simulink model "fazova_trajektorie"  (R2018a)
settings: Solver=VariableStepAuto  StartTime=0.0  StopTime=20  RelTol=1e-3
values from neighbouring files (symbols this model uses):
  K2 = 0.02    [init.m]
  Kz = 20    [init.m]
  T = 2    [init.m]
  Ul = 10    [init.m]
  Un = 25    [init.m]
  w0 = w(i)    [init.m]
settings Model: Creator=vejvarm  LastModifiedBy=Martin

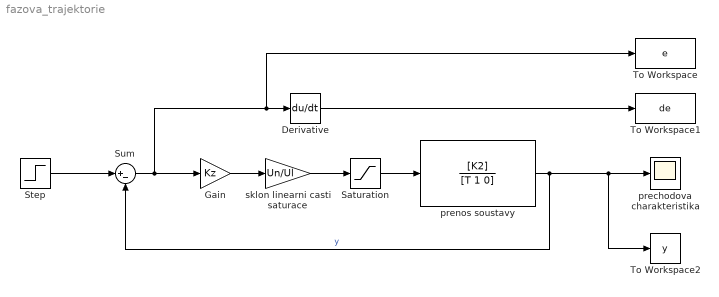
== system fazova_trajektorie ==
  Derivative : Derivative
  Gain : Gain  Gain=Kz
  Saturation : Saturate  UpperLimit=Un  LowerLimit=-Un
  Step : Step  Time=0  After=w0  SampleTime=0
  Sum : Sum  Inputs=|+-
  To Workspace : ToWorkspace  VariableName=e  SaveFormat=Structure With Time  SampleTime=-1
  To Workspace1 : ToWorkspace  VariableName=de  SaveFormat=Structure With Time  SampleTime=-1
  To Workspace2 : ToWorkspace  VariableName=y  SaveFormat=Structure With Time  SampleTime=-1
  prechodova charakteristika : Scope
  prenos soustavy : TransferFcn  Numerator=[K2]  Denominator=[T 1 0]
  sklon linearni casti saturace : Gain  Gain=Un/Ul
  wires:
  Step/1 -> Sum/1
  Sum/1 -> To Workspace/1, Derivative/1, Gain/1
  Gain/1 -> sklon linearni casti saturace/1
  Saturation/1 -> prenos soustavy/1
  prenos soustavy/1 -> Sum/2, To Workspace2/1, prechodova charakteristika/1  "y"
  sklon linearni casti saturace/1 -> Saturation/1
  Derivative/1 -> To Workspace1/1
